simulink model "s0527"  (Simulink 7.0)
settings: Solver=ode45  SolverMode=SingleTasking  StartTime=0.0  StopTime=100  MaxStep=.1  RelTol=1e-3  AbsTol=1e-6
values from neighbouring files (symbols this model uses):
  Kpr = 10    [m0108d.m]    (also in m0109b.m = 1; m0113c.m; m0404Bsp.m = 3)
  Tt = .4    (= 0.4)    [m0108d.m]    (also in m0259.m = 1; m0314.m = 2.13; m0322.m = 0.8; m0326.m = 4)
undefined symbols (not defined in the file or in its folder): Iein, snen, szae, Tn, Tv
libraries: srolib x1
settings Model: Creator=froriep  LastModifiedBy=froriep
settings DataIOCC: LimitDataPoints=off  SaveOutput=off  TimeSaveName=t  SignalLoggingName=sigsOut
settings OptimizationCC: BooleanDataType=off  InlineInvariantSignals=on
settings DebuggingCC: SaveWithParameterizedLinksMsg=none  SignalResolutionControl=TryResolveAllWithWarning  SolverPrmCheckMsg=none  MultiTaskDSMMsg=warning  MultiTaskCondExecSysMsg=none  StrictBusMsg=None
settings HardwareCC: TargetUnknown=on
settings RTWCC: IncludeERTFirstTime=on
settings GRTTargetCC: TargetFcnLib=ansi_tfl_tmw.mat  ModelReferenceCompliant=off  MatFileLogging=off

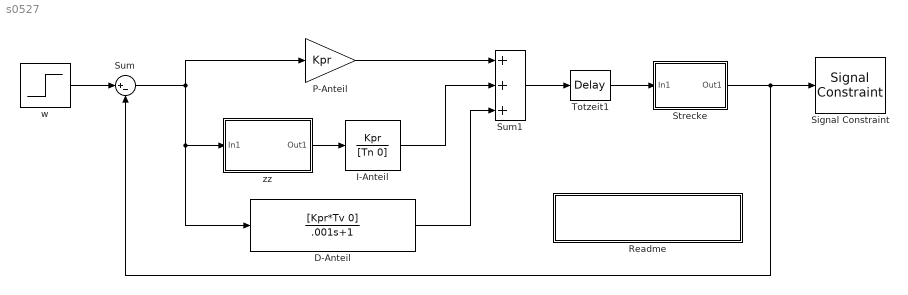
== system s0527 ==
  D-Anteil : TransferFcn  Numerator=[Kpr*Tv 0]  Denominator=[.001 1]
  I-Anteil : TransferFcn  Numerator=Kpr  Denominator=[Tn 0]
  P-Anteil : Gain  Gain=Kpr  ParameterDataType=sfix(16)  ParameterScaling=2^0  OutDataType=sfix(16)  OutScaling=2^0  SaturateOnIntegerOverflow=on
  Readme : Subsystem
      mask Display: disp('Bitte hier doppelklicken')
  Signal Constraint : srolib/Signal Constraint  SystemSampleTime=-1  DialogPosition=[0.47734375 0.056640625 0.45 0.3095703125]  SaveIn=MAT file  SaveAs=s0527_optim.mat  LogID=SRO_DataLog_1  Ylim=[-0.1 1.2]
  Strecke : Subsystem
      mask Display: disp('Gs(s)')
  Sum : Sum  Inputs=|+-  OutDataType=sfix(16)  OutScaling=2^0  SaturateOnIntegerOverflow=on  InputSameDT=on
  Sum1 : Sum  Inputs=+++  OutDataType=sfix(16)  OutScaling=2^0  SaturateOnIntegerOverflow=on  InputSameDT=on
  Totzeit1 : TransportDelay  DelayTime=Tt
  w : Step  Time=0  SampleTime=0  ZeroCross=off
  zz : Subsystem
      mask Display: disp('Schalter')
  wires:
  Sum1/1 -> Totzeit1/1
  Totzeit1/1 -> Strecke/1(In1)
  I-Anteil/1 -> Sum1/2
  zz/1(Out1) -> I-Anteil/1
  Strecke/1(Out1) -> Sum/2, Signal Constraint/1
  D-Anteil/1 -> Sum1/3
  Sum/1 -> P-Anteil/1, D-Anteil/1, zz/1(In1)
  P-Anteil/1 -> Sum1/1
  w/1 -> Sum/1

== system s0527/Readme ==
  note: Die Optimierung wird gestartet, indem man
      | in der Menüleiste "Optimization" auswählt und darin "Start" anklickt.
      | Tuned Parameters: Kpr und Tn
  note: Die Sprungantwort für die Regler-Startwerte wird  eingezeichnet,
      | indem man in der Menuleiste
      | "Plots" und dann "Plot Current Response" anwählt.
  note: Man erhält das Diagramm von Bild 5.27, indem man auf den grünen
      | Block "Signal Constraint" doppelklickt.
      |
      | (Das funktioniert nur, wenn
      | Simulink Response Optimization installiert ist.)

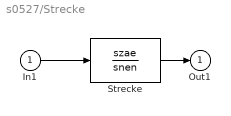
== system s0527/Strecke ==
  In1 : Inport  OutDataType=sfix(16)  OutScaling=2^0
  Strecke : TransferFcn  Numerator=szae  Denominator=snen
  Out1 : Outport  OutDataType=sfix(16)  OutScaling=2^0
  wires:
  In1/1 -> Strecke/1
  Strecke/1 -> Out1/1

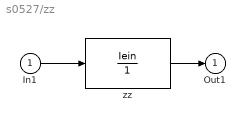
== system s0527/zz ==
  In1 : Inport  OutDataType=sfix(16)  OutScaling=2^0
  zz : TransferFcn  Numerator=Iein  Denominator=1
  Out1 : Outport  OutDataType=sfix(16)  OutScaling=2^0
  wires:
  In1/1 -> zz/1
  zz/1 -> Out1/1
